simulink model "NoEngineController"  (R2025b)
settings: configuration reference "EngFixed10ms" (kept outside this file)
settings Model: DataDictionary=VirtualDynoTemplate.sldd  ModifiedByFormat=The MathWorks, Inc.  Creator=The MathWorks, Inc.  LastModifiedBy=The MathWorks, Inc.
settings ConfigSetRef: SourceName=EngFixed10ms

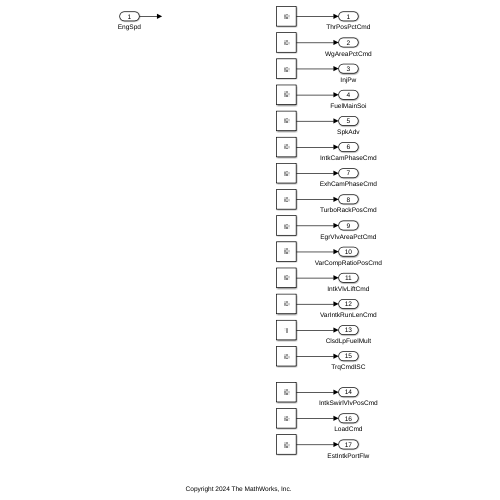
[thumbnail: Simulink's stored preview of the top-level diagram]
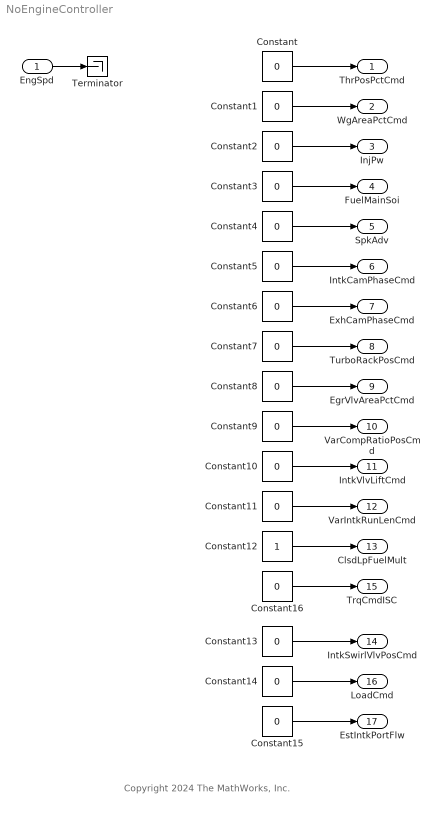
== system NoEngineController ==
  note: Copyright 2024 The MathWorks, Inc.
  EngSpd : Inport  Unit=rpm
  Constant{,1..11,13..16} (16 alike) : Constant  Value=0  SampleTime=-1
  Constant12 : Constant  SampleTime=-1
  Terminator : Terminator
  ThrPosPctCmd : Outport  VectorParamsAs1DForOutWhenUnconnected=off
  WgAreaPctCmd : Outport  Port=2  VectorParamsAs1DForOutWhenUnconnected=off
  InjPw : Outport  Port=3  SampleTime=0.01  VectorParamsAs1DForOutWhenUnconnected=off
  FuelMainSoi : Outport  Port=4  Unit=deg  VectorParamsAs1DForOutWhenUnconnected=off
  SpkAdv : Outport  Port=5  VectorParamsAs1DForOutWhenUnconnected=off
  IntkCamPhaseCmd : Outport  Port=6  VectorParamsAs1DForOutWhenUnconnected=off
  ExhCamPhaseCmd : Outport  Port=7  VectorParamsAs1DForOutWhenUnconnected=off
  TurboRackPosCmd : Outport  Port=8  Unit=1  VectorParamsAs1DForOutWhenUnconnected=off
  EgrVlvAreaPctCmd : Outport  Port=9  Unit=%  VectorParamsAs1DForOutWhenUnconnected=off
  VarCompRatioPosCmd : Outport  Port=10  VectorParamsAs1DForOutWhenUnconnected=off
  IntkVlvLiftCmd : Outport  Port=11  VectorParamsAs1DForOutWhenUnconnected=off
  VarIntkRunLenCmd : Outport  Port=12  VectorParamsAs1DForOutWhenUnconnected=off
  ClsdLpFuelMult : Outport  Port=13  VectorParamsAs1DForOutWhenUnconnected=off
  IntkSwirlVlvPosCmd : Outport  Port=14  VectorParamsAs1DForOutWhenUnconnected=off
  TrqCmdISC : Outport  Port=15  VectorParamsAs1DForOutWhenUnconnected=off
  LoadCmd : Outport  Port=16  VectorParamsAs1DForOutWhenUnconnected=off
  EstIntkPortFlw : Outport  Port=17  VectorParamsAs1DForOutWhenUnconnected=off
  wires:
  Constant8/1 -> EgrVlvAreaPctCmd/1
  Constant4/1 -> SpkAdv/1
  Constant3/1 -> FuelMainSoi/1
  Constant12/1 -> ClsdLpFuelMult/1
  Constant9/1 -> VarCompRatioPosCmd/1
  Constant2/1 -> InjPw/1
  Constant1/1 -> WgAreaPctCmd/1
  Constant5/1 -> IntkCamPhaseCmd/1
  Constant13/1 -> IntkSwirlVlvPosCmd/1
  Constant15/1 -> EstIntkPortFlw/1
  Constant7/1 -> TurboRackPosCmd/1
  Constant6/1 -> ExhCamPhaseCmd/1
  Constant16/1 -> TrqCmdISC/1
  Constant11/1 -> VarIntkRunLenCmd/1
  Constant10/1 -> IntkVlvLiftCmd/1
  Constant14/1 -> LoadCmd/1
  Constant/1 -> ThrPosPctCmd/1
  EngSpd/1 -> Terminator/1
